simulink subsystem "Infrarrojos2"  (R2024b)
settings: Solver=VariableStepAuto  StartTime=0.0  StopTime=10.0  RelTol=1e-3
libraries: arduinolib x2
settings Model: Creator=Laura  LastModifiedBy=Laura

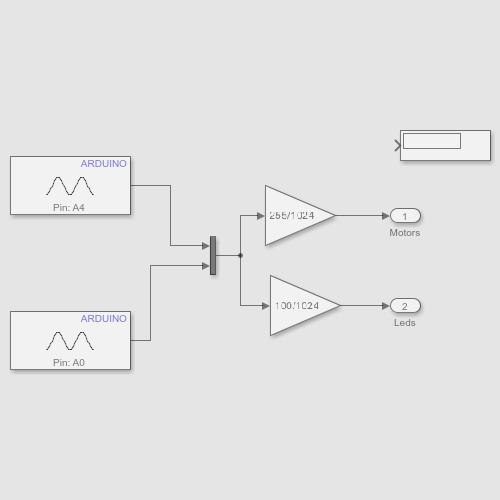
[thumbnail: Simulink's stored preview of the top-level diagram]
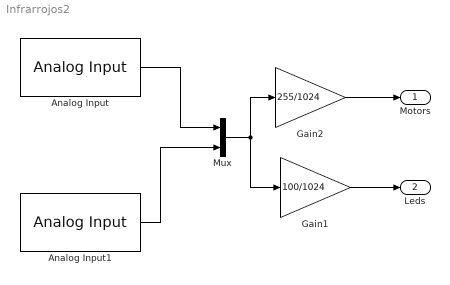
== system Infrarrojos2 ==
  Analog Input : arduinolib/Analog Input  pinNumber=4  ReadResultsOnly=off  ConversionTriggerSource=Software  ExternalTriggerType=uint32( 0 )  OutputDataType=uint16  EnableConversionCompleteNotify=off  EnableOuputStatus=off  SampleTime=-1  blockPlatform=arduino
  Analog Input1 : arduinolib/Analog Input  pinNumber=0  ReadResultsOnly=off  ConversionTriggerSource=Software  ExternalTriggerType=uint32( 0 )  OutputDataType=uint16  EnableConversionCompleteNotify=off  EnableOuputStatus=off  SampleTime=-1  blockPlatform=arduino
  Gain1 : Gain  Gain=100/1024
  Gain2 : Gain  Gain=255/1024
  Mux : Mux  Inputs=2
  Motors : Outport
  Leds : Outport  Port=2
  wires:
  Analog Input/1 -> Mux/1
  Analog Input1/1 -> Mux/2
  Mux/1 -> Gain2/1, Gain1/1
  Gain2/1 -> Motors/1
  Gain1/1 -> Leds/1
